simulink model "BlindSpotLogicSWC"  (R2024b)
settings: Solver=FixedStepDiscrete  StartTime=0.0  StopTime=10.0  FixedStep=0.1  RelTol=1e-3
values from neighbouring files (symbols this model uses):
  TurnSignalStatusType : value not decoded    [BlindSpotDataTypes.sldd]
libraries: sldvlib x2
settings Model: DataDictionary=BlindSpotDataTypes.sldd  Creator=Emir  LastModifiedBy=Emir
settings OptimizationCC: DefaultParameterBehavior=Inlined  EnhancedBackFolding=on  PassReuseOutputArgsAs=Individual arguments  ZeroExternalMemoryAtStartup=off  ZeroInternalMemoryAtStartup=off  OptimizeBlockOrder=speed  DifferentSizesBufferReuse=on  OptimizationCustomize=off  EfficientTunableParamExpr=on
settings DebuggingCC: ParameterTunabilityLossMsg=error
settings SFSimCC: MATLABDynamicMemAlloc=off
settings RTWCC: Description=AUTOSAR  SystemTargetFile=autosar.tlc  GenCodeOnly=on  TemplateMakefile=ert_default_tmf  DataTypeReplacement=CDataTypesFixedWidth
settings CodeAppCC: ForceParamTrailComments=on  IgnoreCustomStorageClasses=off  OperatorAnnotations=on  SimulinkDataObjDesc=on  SFDataObjDesc=on  InsertBlockDesc=on
settings STFCustomTargetCC: TargetLangStandard=C99 (ISO)  MultiwordLength=256  ParMdlRefBuildCompliant=on  CompOptLevelCompliant=on  IncludeMdlTerminateFcn=off  CombineOutputUpdateFcns=on  SuppressErrorStatus=on  ERTCustomFileBanners=on  SupportNonFinite=off  SupportComplex=off  SupportContinuousTime=off  SupportNonInlinedSFcns=off  RemoveResetFunc=on  MATLABClassNameForMDSCustomization=Simulink.SoftwareTarget.ERTCustomization  AutosarCompliant=on  UseToolchainInfoCompliant=on  LookupTableObjectStructAxisOrder=2,1,3,4,...  LUTObjectStructOrderEvenSpacing=Size,Table,Breakpoints  SystemTargetFile=autosar.tlc
settings ERTTargetCC: TargetLangStandard=C99 (ISO)  ConcurrentExecutionCompliant=off  IncludeMdlTerminateFcn=off  SuppressErrorStatus=on  SupportNonFinite=off  SupportComplex=off  ModelStepFunctionPrototypeControlCompliant=off  CPPClassGenCompliant=off  AutosarCompliant=on  LookupTableObjectStructAxisOrder=2,1,3,4,...  LUTObjectStructOrderEvenSpacing=Size,Table,Breakpoints  ERTCustomFileTemplate=example_file_process.tlc  BooleanTrueId=TRUE  BooleanFalseId=FALSE

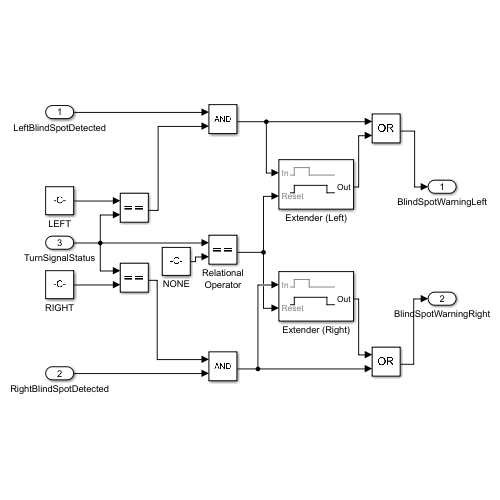
[thumbnail: Simulink's stored preview of the top-level diagram]
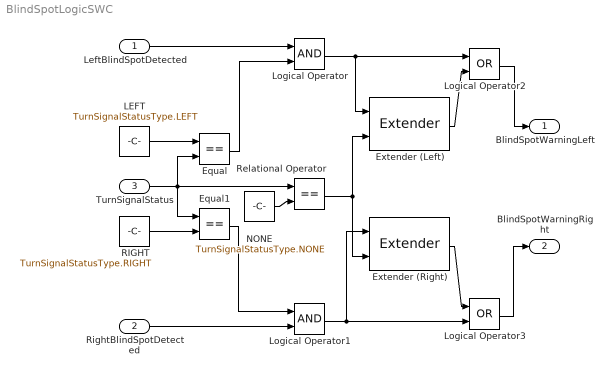
== system BlindSpotLogicSWC ==
  LeftBlindSpotDetected : Inport  OutDataTypeStr=BlindSpotDetectedType
  RightBlindSpotDetected : Inport  Port=2  OutDataTypeStr=BlindSpotDetectedType
  TurnSignalStatus : Inport  Port=3  OutDataTypeStr=Enum: TurnSignalStatusType
  Equal : RelationalOperator  Operator===  OutDataTypeStr=boolean  RndMeth=Simplest  InputSameDT=off
  Equal1 : RelationalOperator  Operator===  OutDataTypeStr=boolean  RndMeth=Simplest  InputSameDT=off
  Extender (Left) : sldvlib/Temporal Operators/Extender  reset=on  ext_type=Finite  out_hold=20
  Extender (Right) : sldvlib/Temporal Operators/Extender  reset=on  ext_type=Finite  out_hold=20
  LEFT : Constant  Value=TurnSignalStatusType.LEFT  OutDataTypeStr=Enum: TurnSignalStatusType
  Logical Operator : Logic  AllPortsSameDT=off  OutDataTypeStr=boolean
  Logical Operator1 : Logic  AllPortsSameDT=off  OutDataTypeStr=boolean
  Logical Operator2 : Logic  Operator=OR  AllPortsSameDT=off  OutDataTypeStr=boolean
  Logical Operator3 : Logic  Operator=OR  AllPortsSameDT=off  OutDataTypeStr=boolean
  NONE : Constant  Value=TurnSignalStatusType.NONE  OutDataTypeStr=Enum: TurnSignalStatusType
  RIGHT : Constant  Value=TurnSignalStatusType.RIGHT  OutDataTypeStr=Enum: TurnSignalStatusType
  Relational Operator : RelationalOperator  Operator===  OutDataTypeStr=boolean  RndMeth=Simplest  InputSameDT=off
  BlindSpotWarningLeft : Outport  OutDataTypeStr=BlindSpotWarningType
  BlindSpotWarningRight : Outport  Port=2  OutDataTypeStr=BlindSpotWarningType
  wires:
  TurnSignalStatus/1 -> Equal/2, Relational Operator/1, Equal1/1
  LEFT/1 -> Equal/1
  RIGHT/1 -> Equal1/2
  RightBlindSpotDetected/1 -> Logical Operator1/2
  LeftBlindSpotDetected/1 -> Logical Operator/1
  Equal/1 -> Logical Operator/2
  Equal1/1 -> Logical Operator1/1
  Logical Operator/1 -> Extender (Left)/1, Logical Operator2/1
  Logical Operator2/1 -> BlindSpotWarningLeft/1
  Logical Operator1/1 -> Logical Operator3/2, Extender (Right)/1
  Logical Operator3/1 -> BlindSpotWarningRight/1
  Extender (Left)/1 -> Logical Operator2/2
  NONE/1 -> Relational Operator/2
  Relational Operator/1 -> Extender (Right)/2, Extender (Left)/2
  Extender (Right)/1 -> Logical Operator3/1
